simulink library "pmm"  (R2021b)
settings: Solver=VariableStepAuto  StartTime=0.0  StopTime=10.0  RelTol=1e-3
undefined symbols (not defined in the file or in its folder): ENUM_ACMAINRLYSTS_OPEN, ENUM_ACPRECHRGRLYSTS_OPEN, ENUM_B2VRLYSTA_OPEN, ENUM_BMSHVSTS_HVOPEN, ENUM_BRAKEPEDAL_RELEASED, ENUM_CACRLYDEM_CLOSE, ENUM_CACRLYSTS_OPEN, ENUM_CHRGFAULT_ACRLYFAIL, ENUM_CHRGFAULT_BCUHVFAIL, ENUM_CHRGFAULT_BCUNEGFAIL, ENUM_CHRGFAULT_BCUTIMEOUT, ENUM_CHRGFAULT_DCDCENABLE, ENUM_CHRGFAULT_DCDCRLYFAIL, ENUM_CHRGFAULT_HVILFAIL, ENUM_CHRGFAULT_PDUHVFAIL, ENUM_CHRGFAULT_RLYCHKFAIL, ENUM_DCDCEACPCURLYSTA_CLOSED, ENUM_DCDCEACPCURLYSTA_FAILTOCLOSE, ENUM_DCDCEACPCURLYSTA_OPEN, ENUM_DCDCEACPCURLYSTA_WELDED, ENUM_DCDCENABLESTS_READY, ENUM_DCDCRLYSTS_OPEN, ENUM_EHPSRLYDEM_CLOSE, ENUM_EHPSRLYSTS_OPEN, ENUM_FOGRLYENCMD_DISABLE, ENUM_GEARACTUALPOSN_D, ENUM_HVPWROFFREQ_POWEROFF, ENUM_KEYSTATUS_OFF, ENUM_KEYSTATUS_ON, ENUM_KEYSTATUS_START, ENUM_LOWBATTVOLTAGE_NORMAL, ENUM_LOWBATTVOLTAGE_POWERDOWN, ENUM_LOWBATTVOLTAGE_POWERUP, ENUM_MCUHVLOOP_POWEROFF, ENUM_MCUHVLOOPSTS_OPEN, ENUM_MCUMAINRLYSTS_OPEN, ENUM_MCUPRECHRGRLYSTS_OPEN, ENUM_PDFAULT_ACRLYOPEN, ENUM_PDFAULT_BCUDISABLE, ENUM_PDFAULT_DCDCDISABLE, ENUM_PDFAULT_DCDCRLYOPEN, ENUM_PDFAULT_EACDISABLE, ENUM_PDFAULT_EACRLYOPEN, ENUM_PDFAULT_EHPSDISABLE, ENUM_PDFAULT_EHPSRLYOPEN, ENUM_PDFAULT_MCUDISABLE, ENUM_PDFAULT_MCUDISCHRG, ENUM_PDFAULT_MCURLYOPEN, ENUM_PEUSELFCHKSTS_NOFAULT, ENUM_PLUGINSTS_NOPLUGIN, ENUM_PLUGINSTS_PLUGIN, ENUM_PMMMODE_DRIVE, ENUM_PMMMODE_LVBATCHRG, ENUM_PUSTATE_DCDCENABLE, ENUM_PUSTATE_EACPRESCHECK, ENUM_PUSTATE_EHPSENABLE, ENUM_PUSTATE_MCUENABLE, ENUM_PUSTATE_PDUMCURLYCLOSED, ENUM_PUSTATE_POWERUPFAIL, ENUM_TARGETGEAR_REVERSE ... (+126)
libraries: hcu_lib x45, simulink x5, ddm x1, dsc x1
(part 1 of 7)
settings Model: Creator=13615  LastModifiedBy=zack
settings SolverCC: AlgebraicLoopSolver=TrustRegion
settings DataIOCC: SaveFormat=Array  SignalLoggingSaveFormat=ModelDataLogs  ReturnWorkspaceOutputs=off
settings OptimizationCC: BlockReduction=off  BooleanDataType=off
settings DebuggingCC: SaveWithParameterizedLinksMsg=none  UnderspecifiedInitializationDetection=Classic  MergeDetectMultiDrivingBlocksExec=none  SignalResolutionControl=TryResolveAllWithWarning  SFMachineParentedDataDiag=warning  ArithmeticOperatorsInVariantConditions=warning
settings HardwareCC: TargetUnknown=on
settings ModelReferenceCC: PropagateSignalLabelsOutOfModel=off
settings SFSimCC: SimUseLocalCustomCode=off  CustomCodeUndefinedFunction=UseInterfaceOnly
settings RTWCC: RTWUseLocalCustomCode=off
settings ConfigComp: CovMetricSettings=dw  CovSaveCumulativeToWorkspaceVar=on  CovSaveSingleToWorkspaceVar=on

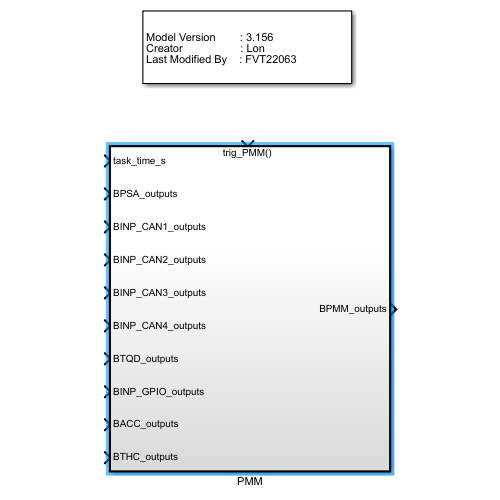
[thumbnail: Simulink's stored preview of the top-level diagram]
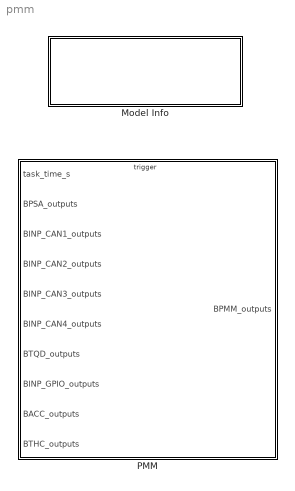
== system pmm ==
  Model Info : Subsystem  LoadFcn=slcm LoadBlock;  InitFcn=slcm('UpdateAllCMBlocksInThisModelInit')  mask(CMBlock){InitialSaveTempField=, InitialBlockCM=None, BlockCM=None, Frame=on, SaveTempField=, DisplayStringWithTags=|, MaskDisplayString=Model Version        : 3.157\nCreator                   : Lon\nLast Modified By    : zack, HorizontalTextAlignment=Left, LeftAlignmentValue=0.02, SourceBlockDiagram=pmm, TagMaxNumber=20, CMTag1=, CMTag2=, CMTag3=, CMTag4=, CMTag5=, CMTag6=, CMTag7=, CMTag8=, CMTag9=, CMTag10=, CMTag11=, CMTag12=, CMTag13=, CMTag14=, CMTag15=, CMTag16=, CMTag17=, CMTag18=, CMTag19=, CMTag20=}
      mask DisplayStringWithTags=|
      | Model Version        : %<ModelVersion>
      | Creator                   : Lon
      | Last Modified By    : %<LastModifiedBy>
      mask help: This block allows revision control information to be displayed within the model.
      settings: CopyFcn=slcm CopyBlock;  DeleteFcn=slcm Cancel;  PostSaveFcn=slcm('UpdateAllCMBlocksInThisModel')  NameChangeFcn=slcm Rename;  OpenFcn=slcm
      mask Display: text(str2num(LeftAlignmentValue), 0.5, MaskDisplayString, 'HorizontalAlignment', HorizontalTextAlignment)
  PMM : Subsystem  TreatAsAtomicUnit=on
      settings: RTWSystemCode=Nonreusable function  RTWFcnNameOpts=Use subsystem name  RTWFileNameOpts=Use subsystem name

== system pmm/Model Info ==
  EmptySubsystem : Subsystem

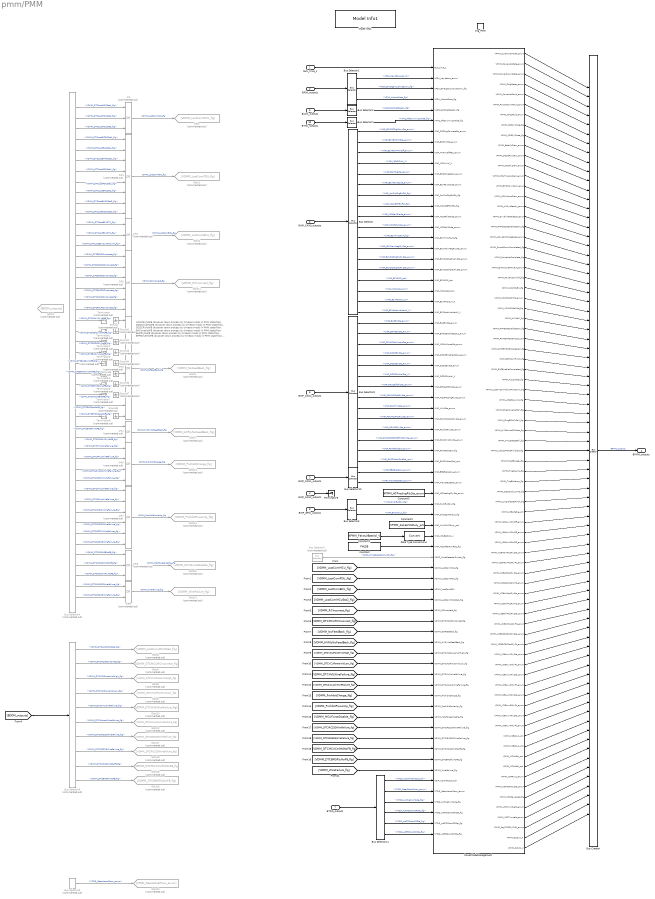
== system pmm/PMM ==
  note: ACHCRlyNoFB do power down process by timeout modul in PMM state flow.
      | DCDCInverNoFB do power down process by timeout modul in PMM state flow.
      | DCDCRlyNoFB do power down process by timeout modul in PMM state flow.
      | EACInverNoFB do power down process by timeout modul in PMM state flow.
      | EACRlyNoFB do power down process by timeout modul in PMM state flow.
      | EHPSInverNoFB do power down process by timeout modul in PMM state flow.
      | EHPSRlyNoFB do power down process by timeout modul in PMM state flow.
      | MCUHVRlyNoFB do power down process by timeout modul in PMM state flow.
      | BMSRlyNoFB do power down process by timeout modul in PMM state flow.
      | MCUIGBNoFB do power down process by timeout modul in PMM state flow.
      | EHPSSpdNOFB do power down process by timeout modul in PMM state flow.
      | Keep relay/inverter closed for driving ability.
  task_time_s : Inport
  BPSA_outputs : Inport  Port=2  OutDataTypeStr=Bus: BPSA_outputs
  BINP_CAN1_outputs : Inport  Port=3  OutDataTypeStr=Bus: BINP_CAN1_outputs
  BINP_CAN2_outputs : Inport  Port=4  OutDataTypeStr=Bus: BHAL_CAN2_outputs
  BINP_CAN3_outputs : Inport  Port=5  OutDataTypeStr=Bus: BINP_CAN3_outputs
  BINP_CAN4_outputs : Inport  Port=6  OutDataTypeStr=Bus: BINP_CAN4_outputs
  BTQD_outputs : Inport  Port=7  OutDataTypeStr=Bus: BTQD_outputs
  BINP_GPIO_outputs : Inport  Port=8  OutDataTypeStr=Bus: BINP_GPIO_outputs
  BACC_outputs : Inport  Port=9  OutDataTypeStr=Bus: BACC_outputs
  BTHC_outputs : Inport  Port=10  OutDataTypeStr=Bus: BTHC_outputs
  trig_PMM : TriggerPort  TriggerType=function-call  VariantControl=(inherit)
  Bus Creator : BusCreator  Inputs=79  OutDataTypeStr=Bus: BPMM_outputs  NonVirtualBus=on
  Bus Selector : BusSelector  OutputSignals=VINP_B2VDCChgConnSta_enum,VINP_B2VBMUHVSta_enum,VINP_B2VRqHVPwrOff_enum,VINP_MCUDCVol_V,VINP_B2VChgSta_enum,VINP_B2VFaultCode_enum,VINP_AtvDisChgEnFbk_flg,VINP_MCUIGBTEnFbk_flg,VINP_MCUFailGrade_enum,VINP_MCUFailCode_enum,VINP_B2VHVILFault_flg,VINP_B2VMainNegRlySta_enum,VINP_B2VDCChgP1RlySta_enum,VINP_B2VDCChgN1RlySta_enum,VINP_B2VSOC_pct,VINP_MotorSpd_rpm,VINP_B2VPackCurr_A,VINP_B2VPackInsideVol_V
  Bus Selector1 : BusSelector  OutputSignals=VPSA_Keystatus_enum,VPSA_EmergencyShutDown_flg,VPSA_AlcLockPass_flg
  Bus Selector10 : BusSelector  OutputSignals=VINP_EBSBrakeSw_enum,VINP_TransReqGear_enum
  Bus Selector11 : BusSelector  OutputSignals=VTQD_VCUTMVehSpd_kph,VTQD_GearActualPosn_enum,VTQD_LVchrgSvrMode_flg,VTQD_ActMDDoorOPSta_flg,VTQD_ActTDDoorOPSta_flg,VTQD_ActFRDoorOPSta_flg
  Bus Selector2 : BusSelector  OutputSignals=VACC_CACPresReady_flg
  Bus Selector3 : BusSelector  Commented=on  OutputSignals=VDSC_WineDetectorSwitch_flg
  Bus Selector4 : BusSelector  Commented=on  OutputSignals=VDMM_DTCLostMCUSta1_flg,VDMM_DTCLostMCUSta2_flg,VDMM_DTCLostMCUSta3_flg,VDMM_DTCLostDCDCSta1_flg,VDMM_DTCLostEACSta1_flg,VDMM_DTCLostEHPSSta1_flg,VDMM_DTCLostPDUSta1_flg,VDMM_DTCLostPDUSta2_flg,VDMM_DTCLostEACSta2_flg,VDMM_DTCLostEHPSSta2_flg,VDMM_DTCLostDCDCSta2_flg,VDMM_DTCLostB2VST1_flg,VDMM_DTCLostB2VST2_flg,VDMM_DTCLostB2VCurrentLimit_flg,VDMM_DTCBCURCIncorrect_flg,VDMM_DTCDCDCRCIncorrect_flg,VDMM_DTCEACRCIncorrect_flg,VDMM_DTCEHPSRCIncorrect_flg,VDMM_DTCMCURCIncorrect_flg,VDMM_DTCPDURCIncorrect_flg,VDMM_DTCACHVRlyNoFB_flg,VDMM_DTCDCDCInverNoFB_flg,VDMM_DTCDCDCRlyNoFB_flg,VDMM_DTCEACInverNoFB_flg,VDMM_DTCEACRlyNoFB_flg,VDMM_DTCEHPSInverNoFB_flg,VDMM_DTCEHPSRlyNoFB_flg,VDMM_DTCMCUIGBNoFB_flg,VDMM_DTCEACSpdNoFB_flg,VDMM_DTCEHPSSpdNoFB_flg,VDMM_DTCBMSRlyNoFB_flg,VDMM_DTCMCUHVRlyNoFB_flg,VDMM_DTCHVILWireFailure_flg,VDMM_DTCAPlusWireFailure_flg,VDMM_DTCAPlusS2VWireFailure_flg,VDMM_DTCIRCS2VWireFailure_flg,VDMM_DTCHVILWireFailure_flg,VDMM_DTCAPlusWireFailure_flg,VDMM_DTCIGNS2VWireFailure_flg,VDMM_DTCIGNS2GWireFailure_flg,VDMM_DTCIRCS2VWireFailure_flg,VDMM_DTCIRCS2GWireFailure_flg,VDMM_DTCMCUIGBNoFB_flg,VDMM_DTCMCUCtrlMdNoFB_flg,VDMM_DTCMCUHVRlyNoFB_flg,VDMM_DTCIGNS2GWireFailure_flg,VDMM_DTCIRCS2GWireFailure_flg
  Bus Selector5 : BusSelector  OutputSignals=VINP_PushButton_flg,VINP_BmsAplus_flg
  Bus Selector6 : BusSelector  Commented=on  OutputSignals=VDMM_DTCLostMCUSta2_flg,VDMM_DTCMCURCIncorrect_flg,VDMM_DTCVCUPowerVolHigh_flg,VDMM_DTCVCUPowerVolLow_flg,VDMM_DTCHVILWireFailure_flg,VDMM_DTCAlcLockWireFailure_flg,VDMM_DTCIGNS2GWireFailure_flg,VDMM_DTCIRCS2GWireFailure_flg,VDMM_DTCMCUCtrlMdNoFB_flg,VDMM_DTCBMSRlyNoFB_flg
  Bus Selector7 : BusSelector  OutputSignals=VTHC_AfterrunningMode_flg
  Bus Selector8 : BusSelector  Commented=on  OutputSignals=VTQD_GearActualPosn_enum
  Bus Selector9 : BusSelector  OutputSignals=VINP_EACEnSta_enum,VINP_EHPSEnSta_enum,VINP_PDUMCUHVLoopSta_enum,VINP_DCDCEnSta_enum,VINP_DCDCEnSta_enum,VINP_DCDCOutVolSta_V,VINP_PDUSelfChkSta_enum,VINP_PDUMCUPreRlySta_enum,VINP_PDUHVILSta_enum,VINP_PDUMCUPosRlySta_enum,VINP_PDUACRlySta_enum,VINP_PDUDCDCEACEHPSRlySta_enum,VINP_ParkBrakeSW_enum,VINP_EHPSMotorSpdSta_rpm
  Constant : Constant  Value=FALSE
  Constant1 : Constant  Value=KPMM_FakeLVBattVol_V
  Constant2 : Constant  Value=KPMM_FakeHVILDuty_pct
  Constant3 : Constant  Value=KPMM_ACPrechrgRlySts_enum
  Data Type Conversion4 : DataTypeConversion
  Goto : Goto  Commented=on  GotoTag=VDMM_LostComMCU_flg
  Goto1 : Goto  Commented=on  GotoTag=VDMM_LostComPDU_flg
  Goto10 : Goto  Commented=on  GotoTag=VDMM_DTCHVILWireFailure_flg
  Goto11 : Goto  Commented=on  GotoTag=VDMM_RCIncorrect_flg
  Goto12 : Goto  Commented=on  GotoTag=VDMM_DTCAlcLockWireFailure_flg
  Goto13 : Goto  Commented=on  GotoTag=VDMM_ProhibitCharge_flg
  Goto14 : Goto  Commented=on  GotoTag=VDMM_ProhibitPowerUp_flg
  Goto15 : Goto  Commented=on  GotoTag=VDMM_MCUForceDisable_flg
  Goto16 : Goto  Commented=on  GotoTag=VDMM_DTCBMSRlyNoFB_flg
  Goto17 : Goto  Commented=on  GotoTag=VDMM_DTCIGNS2GWireFailure_flg
  Goto18 : Goto  Commented=on  GotoTag=VDMM_DTCIRCS2GWireFailure_flg
  Goto19 : Goto  Commented=on  GotoTag=VDMM_DTCMCUCtrlMdNoFB_flg
  Goto2 : Goto  Commented=on  GotoTag=VDMM_LostComBCU_flg
  Goto21 : Goto  Commented=on  GotoTag=VDMM_WireFailure_flg
  Goto22 : Goto  Commented=on  GotoTag=VTQD_GearActualPosn_enum
  Goto3 : Goto  Commented=on  GotoTag=BDDM_outputs
  Goto4 : Goto  Commented=on  GotoTag=VDMM_NoFeedBack_flg
  Goto5 : Goto  Commented=on  GotoTag=VDMM_DTCMCURCIncorrect_flg
  Goto6 : Goto  Commented=on  GotoTag=VDMM_LostComMCUSta2_flg
  Goto7 : Goto  Commented=on  GotoTag=VDMM_HVRlyNoFeedBack_flg
  Goto8 : Goto  Commented=on  GotoTag=VDMM_DTCVCUPowerVolHigh_flg
  Goto9 : Goto  Commented=on  GotoTag=VDMM_DTCVCUPowerVolLow_flg
  Ground{,1..8} (9 alike) : Ground  Commented=on
  Model Info1 : hcu_lib/Model Info1  BlockCM=None  Frame=on  DisplayStringWithTags=|  HorizontalTextAlignment=Left  LeftAlignmentValue=0.02  SourceBlockDiagram=hcu_lib  TagMaxNumber=20
      | Model Version        : %<ModelVersion>
      | Creator                   : %<Creator>
      | Last Modified By    : %<LastModifiedBy>
      settings: SourceProductName=HCU Relative Block Library
  OR : Logic  Commented=on  Operator=OR  Inputs=3  AllPortsSameDT=off  OutDataTypeStr=boolean
  OR1 : Logic  Commented=on  Operator=OR  Inputs=8  AllPortsSameDT=off  OutDataTypeStr=boolean
  OR2 : Logic  Commented=on  Operator=OR  Inputs=3  AllPortsSameDT=off  OutDataTypeStr=boolean
  OR3 : Logic  Commented=on  Operator=OR  Inputs=10  AllPortsSameDT=off  OutDataTypeStr=boolean
  OR4 : Logic  Commented=on  Operator=OR  AllPortsSameDT=off  OutDataTypeStr=boolean
  OR5 : Logic  Commented=on  Operator=OR  Inputs=6  AllPortsSameDT=off  OutDataTypeStr=boolean
  OR6 : Logic  Commented=on  Operator=OR  Inputs=4  AllPortsSameDT=off  OutDataTypeStr=boolean
  OR7 : Logic  Commented=on  Operator=OR  Inputs=6  AllPortsSameDT=off  OutDataTypeStr=boolean
  OR8 : Logic  Commented=on  Operator=OR  Inputs=3  AllPortsSameDT=off  OutDataTypeStr=boolean
  OR9 : Logic  Commented=on  Operator=OR  AllPortsSameDT=off  OutDataTypeStr=boolean
  PowerModeManagement : Subsystem
  Terminator{,1..8} (9 alike) : Terminator  Commented=on
  Terminator9 : Terminator
  BPMM_outputs : Outport  OutDataTypeStr=Bus: BPMM_outputs  VectorParamsAs1DForOutWhenUnconnected=off
  wires:
  Bus Selector11/3 -> PowerModeManagement/70(VTQD_LVchrgSvrMode_flg)  "<VTQD_LVchrgSvrMode_flg>"
  Ground7/1 -> OR3/8
  Bus Selector4/28 -> Terminator7/1  "<VDMM_DTCMCUIGBNoFB_flg>"
  Ground6/1 -> OR3/7
  Bus Selector4/27 -> Terminator6/1  "<VDMM_DTCEHPSRlyNoFB_flg>"
  Ground5/1 -> OR3/6
  Bus Selector4/26 -> Terminator5/1  "<VDMM_DTCEHPSInverNoFB_flg>"
  PowerModeManagement/39(VPMM_HVILDetectFail_flg) -> Bus Creator/39
  Bus Selector4/25 -> Terminator4/1  "<VDMM_DTCEACRlyNoFB_flg>"
  Bus Selector4/24 -> Terminator3/1  "<VDMM_DTCEACInverNoFB_flg>"
  Bus Selector4/23 -> Terminator2/1  "<VDMM_DTCDCDCRlyNoFB_flg>"
  Bus Selector4/22 -> Terminator1/1  "<VDMM_DTCDCDCInverNoFB_flg>"
  Bus Selector4/21 -> Terminator/1  "<VDMM_DTCACHVRlyNoFB_flg>"
  Ground4/1 -> OR3/5
  Ground3/1 -> OR3/4
  Ground2/1 -> OR3/3
  Ground1/1 -> OR3/2
  Ground/1 -> OR3/1
  [VDMM_RCIncorrect_flg] -> PowerModeManagement/52(VDMM_RCIncorrect_flg)
  [BDDM_outputs] -> Bus Selector6/1
  Bus Creator/1 -> BPMM_outputs/1  "BPMM_outputs"
  [VDMM_LostComMCUSta2_flg] -> PowerModeManagement/51(VDMM_LostComMCUSta2_flg)
  [VDMM_LostComBCU_flg] -> PowerModeManagement/50(VDMM_LostComBCU)
  [VDMM_LostComPDU_flg] -> PowerModeManagement/49(VDMM_LostComPDU_flg)
  [VDMM_LostComMCU_flg] -> PowerModeManagement/48(VDMM_LostComMCU_flg)
  OR2/1 -> Goto2/1  "VDMM_LostComBCU_flg"
  Bus Selector4/14 -> OR2/3  "<VDMM_DTCLostB2VCurrentLimit_flg>"
  Bus Selector4/13 -> OR2/2  "<VDMM_DTCLostB2VST2_flg>"
  Bus Selector4/12 -> OR2/1  "<VDMM_DTCLostB2VST1_flg>"
  OR1/1 -> Goto1/1  "VDMM_LostComPDU_flg"
  Bus Selector4/11 -> OR1/8  "<VDMM_DTCLostDCDCSta2_flg>"
  Bus Selector4/10 -> OR1/7  "<VDMM_DTCLostEHPSSta2_flg>"
  Bus Selector4/9 -> OR1/6  "<VDMM_DTCLostEACSta2_flg>"
  Bus Selector4/8 -> OR1/5  "<VDMM_DTCLostPDUSta2_flg>"
  Bus Selector4/7 -> OR1/4  "<VDMM_DTCLostPDUSta1_flg>"
  Bus Selector4/6 -> OR1/3  "<VDMM_DTCLostEHPSSta1_flg>"
  Bus Selector4/5 -> OR1/2  "<VDMM_DTCLostEACSta1_flg>"
  OR/1 -> Goto/1  "VDMM_LostComMCU_flg"
  Bus Selector4/4 -> OR1/1  "<VDMM_DTCLostDCDCSta1_flg>"
  Bus Selector4/3 -> OR/3  "<VDMM_DTCLostMCUSta3_flg>"
  Bus Selector4/2 -> OR/2  "<VDMM_DTCLostMCUSta2_flg>"
  Bus Selector4/1 -> OR/1  "<VDMM_DTCLostMCUSta1_flg>"
  Bus Selector3/1 -> PowerModeManagement/47(VDSC_WineDetectorSwitch_flg)  "<VDSC_WineDetectorSwitch_flg>"
  Bus Selector/14 -> PowerModeManagement/20(VINP_B2VDCChgN1RlySta_enum)  "<VINP_B2VDCChgN1RlySta_enum>"
  Bus Selector/13 -> PowerModeManagement/19(VINP_B2VDCChgP1RlySta_enum)  "<VINP_B2VDCChgP1RlySta_enum>"
  Bus Selector/12 -> PowerModeManagement/18(VINP_B2VMainNegRlySta_enum)  "<VINP_B2VMainNegRlySta_enum>"
  Bus Selector/6 -> PowerModeManagement/12(VINP_B2VFaultCode_enum)  "<VINP_B2VFaultCode_enum>"
  Bus Selector/11 -> PowerModeManagement/17(VINP_B2VHVILFault_flg)  "<VINP_B2VHVILFault_flg>"
  Bus Selector1/2 -> PowerModeManagement/3(VPSA_EmergencyShutDown_flg)  "<VPSA_EmergencyShutDown_flg>"
  Constant/1 -> PowerModeManagement/46(VINP_MCUAfterRunReq_flg)
  Bus Selector/2 -> PowerModeManagement/8(VINP_BMSHVSts_enum)  "<VINP_B2VBMUHVSta_enum>"
  Bus Selector/1 -> PowerModeManagement/7(VINP_DCChrgConnectSts_enum)  "<VINP_B2VDCChgConnSta_enum>"
  Bus Selector/9 -> PowerModeManagement/15(VINP_MCUFailGrade_enum)  "<VINP_MCUFailGrade_enum>"
  Bus Selector/8 -> PowerModeManagement/14(VINP_MCUIGBTEnFbk_flg)  "<VINP_MCUIGBTEnFbk_flg>"
  Bus Selector2/1 -> PowerModeManagement/5(VACC_CACPresReady_flg)  "<VACC_CACPresReady_flg>"
  Bus Selector1/1 -> PowerModeManagement/2(VPSA_Keystatus_enum)  "<VPSA_Keystatus_enum>"
  BPSA_outputs/1 -> Bus Selector1/1
  task_time_s/1 -> PowerModeManagement/1(task_time_s)
  Bus Selector/3 -> PowerModeManagement/9(VINP_HVPwrOffReq_enum)  "<VINP_B2VRqHVPwrOff_enum>"
  Bus Selector/4 -> PowerModeManagement/10(VINP_MCUInVol_V)  "<VINP_MCUDCVol_V>"
  Bus Selector/5 -> PowerModeManagement/11(VINP_BMSChrgStatus_enum)  "<VINP_B2VChgSta_enum>"
  Bus Selector/7 -> PowerModeManagement/13(VINP_AtvDisChgEnFbk_flg)  "<VINP_AtvDisChgEnFbk_flg>"
  [VDMM_DTCMCURCIncorrect_flg] -> PowerModeManagement/53(VDMM_DTCMCURCIncorrect_flg)
  PowerModeManagement/1(VPMM_SysPowerMode_enum) -> Bus Creator/1
  PowerModeManagement/2(VPMM_PowerUpState_enum) -> Bus Creator/2
  PowerModeManagement/3(VPMM_PowerDownState_enum) -> Bus Creator/3
  PowerModeManagement/4(VPMM_ChrgState_enum) -> Bus Creator/4
  PowerModeManagement/5(VPMM_PowerUpFault_enum) -> Bus Creator/5
  PowerModeManagement/6(VPMM_PowerDownFault_enum) -> Bus Creator/6
  PowerModeManagement/7(VPMM_ChrgFault_enum) -> Bus Creator/7
  PowerModeManagement/8(VPMM_IRCRlyClose_flg) -> Bus Creator/8
  PowerModeManagement/9(VPMM_IGNRlyClose_flg) -> Bus Creator/9
  PowerModeManagement/10(VPMM_BattHVDem_enum) -> Bus Creator/10
  PowerModeManagement/11(VPMM_DCDCRlyDem_enum) -> Bus Creator/11
  PowerModeManagement/12(VPMM_CACRlyDem_enum) -> Bus Creator/12
  PowerModeManagement/13(VPMM_MCUHVLoopDem_enum) -> Bus Creator/13
  PowerModeManagement/14(VPMM_EHPSR lyDem_enum) -> Bus Creator/14
  PowerModeManagement/15(VPMM_ACHVLoopDem_enum) -> Bus Creator/15
  PowerModeManagement/16(VPMM_HVSysReady_enum) -> Bus Creator/16
  PowerModeManagement/17(VPMM_DrivelineRelease_enum) -> Bus Creator/17
  PowerModeManagement/18(VPMM_PMMDCDCEnableDem_flg) -> Bus Creator/18
  PowerModeManagement/19(VPMM_ActiveDischargeReq_enum) -> Bus Creator/19
  PowerModeManagement/20(VPMM_PowerDownCompleted_flg) -> Bus Creator/20
  PowerModeManagement/21(VPMM_PowerUpComplete_flg) -> Bus Creator/21
  PowerModeManagement/22(VPMM_ExtTorquePrevent_enum) -> Bus Creator/22
  PowerModeManagement/23(VPMM_PowerUpInhibit_flg) -> Bus Creator/23
  PowerModeManagement/24(VPMM_VCUMCUEn_flg) -> Bus Creator/24
  PowerModeManagement/25(VPMM_VCUMCUCtrlMd_enum) -> Bus Creator/25
  PowerModeManagement/26(VPMM_VCUMCUFailRst_flg) -> Bus Creator/26
  PowerModeManagement/27(VPMM_HVILFail_flg) -> Bus Creator/27
  PowerModeManagement/28(VPMM_PMMEACEnableDem_flg) -> Bus Creator/28
  PowerModeManagement/29(VPMM_PMMEHPSDemSpd_rpm) -> Bus Creator/29
  PowerModeManagement/30(VPMM_PMMEHPSEnableDem_flg) -> Bus Creator/30
  PowerModeManagement/31(VPMM_EHPSIniFinish_flg) -> Bus Creator/31
  PowerModeManagement/32(VPMM_EACEnableCompleted_flg) -> Bus Creator/32
  PowerModeManagement/33(VPMM_AlcLockSta_flg) -> Bus Creator/33
  PowerModeManagement/34(VPMM_LostHVComActivePwrDown_flg) -> Bus Creator/34
  PowerModeManagement/35(VPMM_LVBattLowInd_flg) -> Bus Creator/35
  PowerModeManagement/36(VPMM_ChrgPowerUpFail_flg) -> Bus Creator/36
  PowerModeManagement/37(VPMM_ChrgBCUHVFail_flg) -> Bus Creator/37
  PowerModeManagement/38(VPMM_HVFailureChkPass_flg) -> Bus Creator/38
  Bus Selector4/15 -> OR5/1  "<VDMM_DTCBCURCIncorrect_flg>"
  Bus Selector4/16 -> OR5/2  "<VDMM_DTCDCDCRCIncorrect_flg>"
  Bus Selector4/17 -> OR5/3  "<VDMM_DTCEACRCIncorrect_flg>"
  Bus Selector4/18 -> OR5/4  "<VDMM_DTCEHPSRCIncorrect_flg>"
  Bus Selector4/19 -> OR5/5  "<VDMM_DTCMCURCIncorrect_flg>"
  Bus Selector4/20 -> OR5/6  "<VDMM_DTCPDURCIncorrect_flg>"
  OR5/1 -> Goto11/1  "VDMM_RCIncorrect_flg"
  Bus Selector6/2 -> Goto5/1  "<VDMM_DTCMCURCIncorrect_flg>"
  Bus Selector6/1 -> Goto6/1  "<VDMM_DTCLostMCUSta2_flg>"
  OR3/1 -> Goto4/1  "VDMM_NoFeedBack_flg"
  OR4/1 -> Goto7/1  "VDMM_HVRlyNoFeedBack_flg"
  Bus Selector6/3 -> Goto8/1  "<VDMM_DTCVCUPowerVolHigh_flg>"
  Bus Selector6/4 -> Goto9/1  "<VDMM_DTCVCUPowerVolLow_flg>"
  [VDMM_NoFeedBack_flg] -> PowerModeManagement/54(VDMM_NoFeedBack_flg)
  [VDMM_HVRlyNoFeedBack_flg] -> PowerModeManagement/55(VDMM_HVRlyNoFeedBack_flg)
  [VDMM_DTCVCUPowerVolHigh_flg] -> PowerModeManagement/56(VDMM_DTCVCUPowerVolHigh_flg)
  [VDMM_DTCVCUPowerVolLow_flg] -> PowerModeManagement/57(VDMM_DTCVCUPowerVolLow_flg)
  Bus Selector6/5 -> Goto10/1  "<VDMM_DTCHVILWireFailure_flg>"
  [VDMM_DTCHVILWireFailure_flg] -> PowerModeManagement/58(VDMM_DTCHVILWireFailure_flg)
  [VDMM_DTCAlcLockWireFailure_flg] -> PowerModeManagement/59(VDMM_DTCAlcLockWireFailure_flg)
  Bus Selector6/6 -> Goto12/1  "<VDMM_DTCAlcLockWireFailure_flg>"
  Bus Selector4/33 -> OR6/1  "<VDMM_DTCHVILWireFailure_flg>"
  Bus Selector4/34 -> OR6/2  "<VDMM_DTCAPlusWireFailure_flg>"
  Bus Selector4/35 -> OR6/3  "<VDMM_DTCAPlusS2VWireFailure_flg>"
  Bus Selector4/36 -> OR6/4  "<VDMM_DTCIRCS2VWireFailure_flg>"
  OR6/1 -> Goto13/1  "VDMM_ProhibitCharge_flg"
  [VDMM_ProhibitCharge_flg] -> PowerModeManagement/60(VDMM_ProhibitCharge_flg)
  Bus Selector4/42 -> OR7/6  "<VDMM_DTCIRCS2GWireFailure_flg>"
  Bus Selector4/41 -> OR7/5  "<VDMM_DTCIRCS2VWireFailure_flg>"
  Bus Selector4/40 -> OR7/4  "<VDMM_DTCIGNS2GWireFailure_flg>"
  Bus Selector4/39 -> OR7/3  "<VDMM_DTCIGNS2VWireFailure_flg>"
  Bus Selector4/38 -> OR7/2  "<VDMM_DTCAPlusWireFailure_flg>"
  Bus Selector4/37 -> OR7/1  "<VDMM_DTCHVILWireFailure_flg>"
  OR7/1 -> Goto14/1  "VDMM_ProhibitPowerUp_flg"
  [VDMM_ProhibitPowerUp_flg] -> PowerModeManagement/61(VDMM_ProhibitPowerUp_flg)
  OR8/1 -> Goto15/1  "VDMM_MCUForceDisable_flg"
  [VDMM_MCUForceDisable_flg] -> PowerModeManagement/62(VDMM_MCUForceDisable_flg)
  Bus Selector4/43 -> OR8/1  "<VDMM_DTCMCUIGBNoFB_flg>"
  Bus Selector4/44 -> OR8/2  "<VDMM_DTCMCUCtrlMdNoFB_flg>"
  Bus Selector6/7 -> Goto17/1  "<VDMM_DTCIGNS2GWireFailure_flg>"
  Bus Selector6/8 -> Goto18/1  "<VDMM_DTCIRCS2GWireFailure_flg>"
  [VDMM_DTCIRCS2GWireFailure_flg] -> PowerModeManagement/63(VDMM_DTCIRCS2GWireFailure_flg)
  [VDMM_DTCIGNS2GWireFailure_flg] -> PowerModeManagement/64(VDMM_DTCIGNS2GWireFailure_flg)
  Bus Selector6/9 -> Goto19/1  "<VDMM_DTCMCUCtrlMdNoFB_flg>"
  [VDMM_DTCMCUCtrlMdNoFB_flg] -> PowerModeManagement/65(VDMM_DTCMCUCtrlMdNoFB_flg)
  Bus Selector4/29 -> OR3/9  "<VDMM_DTCEACSpdNoFB_flg>"
  Bus Selector4/31 -> OR4/1  "<VDMM_DTCBMSRlyNoFB_flg>"
  Bus Selector4/32 -> OR4/2  "<VDMM_DTCMCUHVRlyNoFB_flg>"
  Bus Selector4/45 -> OR8/3  "<VDMM_DTCMCUHVRlyNoFB_flg>"
  Bus Selector6/10 -> Goto16/1  "<VDMM_DTCBMSRlyNoFB_flg>"
  [VDMM_DTCBMSRlyNoFB_flg] -> PowerModeManagement/66(VDMM_DTCBMSRlyNoFB_flg)
  Bus Selector4/30 -> Terminator8/1  "<VDMM_DTCEHPSSpdNoFB_flg>"
  Ground8/1 -> OR3/10
  Bus Selector4/46 -> OR9/1  "<VDMM_DTCIGNS2GWireFailure_flg>"
  Bus Selector4/47 -> OR9/2  "<VDMM_DTCIRCS2GWireFailure_flg>"
  OR9/1 -> Goto21/1  "VDMM_WireFailure_flg"
  [VDMM_WireFailure_flg] -> PowerModeManagement/67(VDMM_WireFailure_flg)
  Bus Selector/15 -> PowerModeManagement/21(VINP_B2VSOC_pct)  "<VINP_B2VSOC_pct>"
  PowerModeManagement/40(VPMM_LVChrgPreActFinished_flg) -> Bus Creator/40
  PowerModeManagement/41(VPMM_TrigRBuzeer_flg) -> Bus Creator/41
  PowerModeManagement/42(VPMM_TrigRLamp_flg) -> Bus Creator/42
  PowerModeManagement/43(VPMM_TrigBrkLamp_flg) -> Bus Creator/43
  PowerModeManagement/44(VPMM_DCDCVolLowTO_flg) -> Bus Creator/44
  Bus Selector/16 -> PowerModeManagement/22(VINP_MotorSpd_rpm)  "<VINP_MotorSpd_rpm>"
  PowerModeManagement/45(VPMM_LongIdleDetFinsh_flg) -> Bus Creator/45
  Bus Selector8/1 -> Goto22/1  "<VTQD_GearActualPosn_enum>"
  Bus Selector11/2 -> PowerModeManagement/69(VTQD_GearActualPosn_enum)  "<VTQD_GearActualPosn_enum>"
  Bus Selector11/4 -> PowerModeManagement/71(VTQD_ActMDDoorOPSta_flg)  "<VTQD_ActMDDoorOPSta_flg>"
  Bus Selector11/5 -> PowerModeManagement/72(VTQD_ActTDDoorOPSta_flg)  "<VTQD_ActTDDoorOPSta_flg>"
  Bus Selector11/6 -> PowerModeManagement/73(VTQD_ActFRDoorOPSta_flg)  "<VTQD_ActFRDoorOPSta_flg>"
  BINP_CAN3_outputs/1 -> Bus Selector/1
  Bus Selector/10 -> PowerModeManagement/16(VINP_MCUFailCode_enum)  "<VINP_MCUFailCode_enum>"
  BINP_CAN4_outputs/1 -> Bus Selector9/1
  Bus Selector9/3 -> PowerModeManagement/27(VINP_MCUHVLoopSts_enum)  "<VINP_PDUMCUHVLoopSta_enum>"
  Bus Selector9/4 -> PowerModeManagement/28(VINP_DCDCEnableStstus_enum)  "<VINP_DCDCEnSta_enum>"
  Bus Selector9/6 -> PowerModeManagement/30(VINP_DCDCOutVol_V)  "<VINP_DCDCOutVolSta_V>"
  Bus Selector9/7 -> PowerModeManagement/31(VINP_PEUSelfChkSts_enum)  "<VINP_PDUSelfChkSta_enum>"
  Bus Selector9/8 -> PowerModeManagement/32(VINP_MCUPrechrgRlySts_enum)  "<VINP_PDUMCUPreRlySta_enum>"
  Bus Selector9/9 -> PowerModeManagement/33(VINP_HVILSta_enum)  "<VINP_PDUHVILSta_enum>"
  BINP_CAN1_outputs/1 -> Bus Selector10/1
  Constant2/1 -> PowerModeManagement/44(VINP_HVILPWMDuty_pct)
  Bus Selector9/10 -> PowerModeManagement/34(VINP_PDUMCUPosRlySta_enum)  "<VINP_PDUMCUPosRlySta_enum>"
  Bus Selector9/11 -> PowerModeManagement/35(VINP_PDUACRlySta_enum)  "<VINP_PDUACRlySta_enum>"
  Bus Selector9/5 -> PowerModeManagement/29(VINP_DCDCEnSta_enum)  "<VINP_DCDCEnSta_enum>"
  Bus Selector9/2 -> PowerModeManagement/26(VINP_EHPSEnableStstus_enum)  "<VINP_EHPSEnSta_enum>"
  Bus Selector9/1 -> PowerModeManagement/25(VINP_EACEnSta_enum)  "<VINP_EACEnSta_enum>"
  Data Type Conversion4/1 -> PowerModeManagement/45(VINP_VCUBattVol_v)
  Constant1/1 -> Data Type Conversion4/1
  Bus Selector10/1 -> PowerModeManagement/39(VINP_EBSBrakeSw_enum)  "<VINP_EBSBrakeSw_enum>"
  BINP_CAN2_outputs/1 -> Terminator9/1
  Constant3/1 -> PowerModeManagement/41(VINP_ACPrechrgRlySts_enum)
  Bus Selector9/13 -> PowerModeManagement/37(VINP_ParkBrakeSW_flg)  "<VINP_ParkBrakeSW_enum>"
  Bus Selector9/12 -> PowerModeManagement/36(VINP_PDU3in1RlySta_enum)  "<VINP_PDUDCDCEACEHPSRlySta_enum>"
  PowerModeManagement/46(VPMM_V2BLifeSig_cnt) -> Bus Creator/46
  PowerModeManagement/47(VPMM_V2BAux1OnOff_enum) -> Bus Creator/47
  PowerModeManagement/48(VPMM_V2BAux2OnOff_enum) -> Bus Creator/48
  PowerModeManagement/49(VPMM_V2BAux3OnOff_enum) -> Bus Creator/49
  PowerModeManagement/50(VPMM_V2BMainPosRlySta_enum) -> Bus Creator/50
  PowerModeManagement/51(VPMM_V2BMainPosRlyFit_enum) -> Bus Creator/51
  PowerModeManagement/52(VPMM_V2BACPosRlySta_enum) -> Bus Creator/52
  PowerModeManagement/53(VPMM_V2BACPosRlyFit_enum) -> Bus Creator/53
  PowerModeManagement/54(VPMM_V2BAirPosRlySta_enum) -> Bus Creator/54
  PowerModeManagement/55(VPMM_V2BAirPosRlyFit_enum) -> Bus Creator/55
  PowerModeManagement/56(VPMM_V2BOilrPosRlySta_enum) -> Bus Creator/56
  PowerModeManagement/57(VPMM_V2BOilPosRlyFit_enum) -> Bus Creator/57
  PowerModeManagement/58(VPMM_V2BDCDCPosRlySta_enum) -> Bus Creator/58
  PowerModeManagement/59(VPMM_V2BDCDCPosRlyFit_enum) -> Bus Creator/59
  PowerModeManagement/60(VPMM_V2BAux1RlySta_enum) -> Bus Creator/60
  PowerModeManagement/61(VPMM_V2BAux1RlyFit_enum) -> Bus Creator/61
  PowerModeManagement/62(VPMM_V2BAux2RlySta_enum) -> Bus Creator/62
  PowerModeManagement/63(VPMM_V2BAux2RlyFit_enum) -> Bus Creator/63
  PowerModeManagement/64(VPMM_V2BAux3RlySta_enum) -> Bus Creator/64
  PowerModeManagement/65(VPMM_V2BAux3RlyFit_enum) -> Bus Creator/65
  PowerModeManagement/66(VPMM_V2BAux4RlySta_enum) -> Bus Creator/66
  PowerModeManagement/67(VPMM_V2BAux4RlyFit_enum) -> Bus Creator/67
  PowerModeManagement/68(VPMM_V2BRsv1_cnt) -> Bus Creator/68
  PowerModeManagement/69(VPMM_V2BRsv2_cnt) -> Bus Creator/69
  PowerModeManagement/70(VPMM_VCULife1_cnt) -> Bus Creator/70
  PowerModeManagement/71(VPMM_VCULife2_cnt) -> Bus Creator/71
  PowerModeManagement/72(VPMM_VSPFunc_enum) -> Bus Creator/72
  PowerModeManagement/73(VPMM_VSPIGNKeySta_enum) -> Bus Creator/73
  PowerModeManagement/74(VPMM_VSPReversed_flg) -> Bus Creator/74
  PowerModeManagement/75(VPMM_VSPTurnRight_enum) -> Bus Creator/75
  PowerModeManagement/76(VPMM_VSPTurnLeft_enum) -> Bus Creator/76
  Bus Selector1/3 -> PowerModeManagement/4(VPSA_AlcLockPass_flg)  "<VPSA_AlcLockPass_flg>"
  PowerModeManagement/77(VPMM_FogTMSRlyCMD_enum) -> Bus Creator/77
  Bus Selector10/2 -> PowerModeManagement/40(VINP_TransReqGear_enum)  "<VINP_TransReqGear_enum>"
  PowerModeManagement/78(VPMM_DCCurr_A) -> Bus Creator/78
  PowerModeManagement/79(VPMM_DCVol_V) -> Bus Creator/79
  BTQD_outputs/1 -> Bus Selector11/1
  Bus Selector11/1 -> PowerModeManagement/68(VDIP_VCUVehSpd_kph)  "<VTQD_VCUTMVehSpd_kph>"
  BINP_GPIO_outputs/1 -> Bus Selector5/1
  Bus Selector5/1 -> PowerModeManagement/42(VINP_PushButton_flg)  "<VINP_PushButton_flg>"
  Bus Selector5/2 -> PowerModeManagement/43(VINP_ChargeWakeup_flg)  "<VINP_BmsAplus_flg>"
  Bus Selector/17 -> PowerModeManagement/23(VINP_B2VPackCurr_A)  "<VINP_B2VPackCurr_A>"
  Bus Selector/18 -> PowerModeManagement/24(VINP_B2VPackInsideVol_V)  "<VINP_B2VPackInsideVol_V>"
  BACC_outputs/1 -> Bus Selector2/1
  Bus Selector9/14 -> PowerModeManagement/38(VINP_EHPSMotorSpd_rpm)  "<VINP_EHPSMotorSpdSta_rpm>"
  BTHC_outputs/1 -> Bus Selector7/1
  Bus Selector7/1 -> PowerModeManagement/6(VTHC_AfterrunningMode_flg)  "<VTHC_AfterrunningMode_flg>"

== system pmm/Model Info/EmptySubsystem ==
